simulink model "SimulinkForEQ"  (R2021b)
settings: Solver=VariableStepAuto  StartTime=0.0  StopTime=inf  RelTol=1e-3
libraries: dspfdesign x5, dspmathops x5, dspsnks4 x1, dspvision x1
settings Model: PacingRate=100  Creator=DSP  LastModifiedBy=DSP

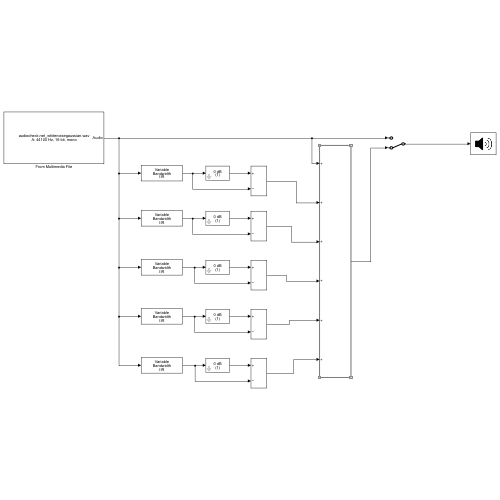
[thumbnail: Simulink's stored preview of the top-level diagram]
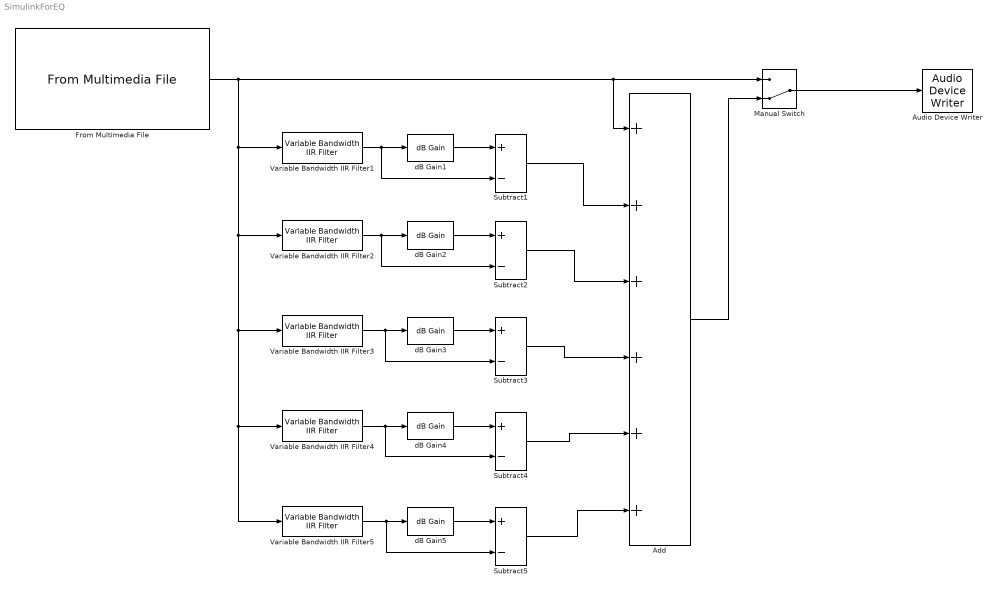
== system SimulinkForEQ ==
  Add : Sum  Inputs=++++++
  Audio Device Writer : dspsnks4/Audio Device Writer  Driver=DirectSound  Device=Default  InheritSampleRate=on  SampleRate=44100  BitDepth=16-bit integer  BufferSize=4096  NumBuffers=10  DefaultOutputChannelMapping=on  OutputChannelMapping=1:2  OutputNumUnderrunSamples=off  DriverIdx=1  DeviceWarnFlag=''
  From Multimedia File : dspvision/From Multimedia File  inputFilename=D:\Jing Sheng\my equalizer\audiocheck.net_whitenoisegaussian.wav  readRange=[1 Inf]  loop=on  numPlays=inf  outputStreams=Audio only  videoDataType=single  audioDataType=double  inheritSampleTime=on  userDefinedSampleTime=1/30  noAudioOutput=off  isIntensityVideo=off  fourcc=RGB  colorVideoFormat=Separate color signals  outputEOF=off  dataOrg=Column-major  audioFrameSize=1024  computeAudioFrameSize=off  outSamplingMode=Sample based
  Manual Switch : ManualSwitch  CurrentSetting=0
  Subtract{1..5} (5 alike) : Sum  Inputs=+-
  Variable Bandwidth IIR Filter1 : dspfdesign/Variable Bandwidth IIR Filter  FilterType=Bandpass  FilterOrder=8  PassbandFrequencyPort=off  PassbandFrequency=512  CenterFrequencyPort=off  CenterFrequency=freq1  BandwidthPort=off  Bandwidth=bw1  PassbandRipple=1  StopbandAttenuation=60  InheritSampleRate=off  SampleRate=44100  SimulateUsing=Code generation
      settings: SourceProductBaseCode=DS
  Variable Bandwidth IIR Filter2 : dspfdesign/Variable Bandwidth IIR Filter  FilterType=Bandpass  FilterOrder=8  PassbandFrequencyPort=off  PassbandFrequency=512  CenterFrequencyPort=off  CenterFrequency=freq2  BandwidthPort=off  Bandwidth=bw2  PassbandRipple=1  StopbandAttenuation=60  InheritSampleRate=off  SampleRate=44100  SimulateUsing=Code generation
      settings: SourceProductBaseCode=DS
  Variable Bandwidth IIR Filter3 : dspfdesign/Variable Bandwidth IIR Filter  FilterType=Bandpass  FilterOrder=8  PassbandFrequencyPort=off  PassbandFrequency=512  CenterFrequencyPort=off  CenterFrequency=freq3  BandwidthPort=off  Bandwidth=bw3  PassbandRipple=1  StopbandAttenuation=60  InheritSampleRate=off  SampleRate=44100  SimulateUsing=Code generation
      settings: SourceProductBaseCode=DS
  Variable Bandwidth IIR Filter4 : dspfdesign/Variable Bandwidth IIR Filter  FilterType=Bandpass  FilterOrder=8  PassbandFrequencyPort=off  PassbandFrequency=512  CenterFrequencyPort=off  CenterFrequency=freq4  BandwidthPort=off  Bandwidth=bw4  PassbandRipple=1  StopbandAttenuation=60  InheritSampleRate=off  SampleRate=44100  SimulateUsing=Code generation
      settings: SourceProductBaseCode=DS
  Variable Bandwidth IIR Filter5 : dspfdesign/Variable Bandwidth IIR Filter  FilterType=Bandpass  FilterOrder=8  PassbandFrequencyPort=off  PassbandFrequency=512  CenterFrequencyPort=off  CenterFrequency=freq5  BandwidthPort=off  Bandwidth=bw5  PassbandRipple=1  StopbandAttenuation=60  InheritSampleRate=off  SampleRate=44100  SimulateUsing=Code generation
      settings: SourceProductBaseCode=DS
  dB Gain1 : dspmathops/dB Gain  dB=gain1  intype=Amplitude
      settings: SourceProductBaseCode=DS
  dB Gain2 : dspmathops/dB Gain  dB=gain2  intype=Amplitude
      settings: SourceProductBaseCode=DS
  dB Gain3 : dspmathops/dB Gain  dB=gain3  intype=Amplitude
      settings: SourceProductBaseCode=DS
  dB Gain4 : dspmathops/dB Gain  dB=gain4  intype=Amplitude
      settings: SourceProductBaseCode=DS
  dB Gain5 : dspmathops/dB Gain  dB=gain5  intype=Amplitude
      settings: SourceProductBaseCode=DS
  wires:
  Manual Switch/1 -> Audio Device Writer/1
  Variable Bandwidth IIR Filter1/1 -> Subtract1/2, dB Gain1/1
  Variable Bandwidth IIR Filter2/1 -> Subtract2/2, dB Gain2/1
  Variable Bandwidth IIR Filter3/1 -> Subtract3/2, dB Gain3/1
  Add/1 -> Manual Switch/2
  dB Gain1/1 -> Subtract1/1
  Subtract1/1 -> Add/2
  dB Gain2/1 -> Subtract2/1
  dB Gain3/1 -> Subtract3/1
  Subtract2/1 -> Add/3
  Subtract3/1 -> Add/4
  From Multimedia File/1 -> Add/1, Manual Switch/1, Variable Bandwidth IIR Filter5/1, Variable Bandwidth IIR Filter4/1, Variable Bandwidth IIR Filter3/1, Variable Bandwidth IIR Filter2/1, Variable Bandwidth IIR Filter1/1
  Variable Bandwidth IIR Filter4/1 -> Subtract4/2, dB Gain4/1
  Variable Bandwidth IIR Filter5/1 -> Subtract5/2, dB Gain5/1
  dB Gain4/1 -> Subtract4/1
  dB Gain5/1 -> Subtract5/1
  Subtract4/1 -> Add/5
  Subtract5/1 -> Add/6
